simulink subsystem "electric_valva"  (R2022b)
settings: Solver=VariableStepAuto  StartTime=0.0  StopTime=10.0  RelTol=1e-3
values from neighbouring files (symbols this model uses):
  K = 6    [valva_run.m]
  L = 0.005    [valva_run.m]
  R = 3    [valva_run.m]
undefined symbols (not defined in the file or in its folder): magnitude
settings Model: Creator=rus_d  LastModifiedBy=rus_d

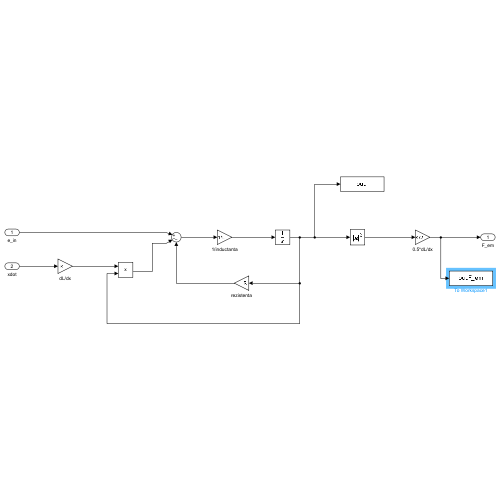
[thumbnail: Simulink's stored preview of the top-level diagram]
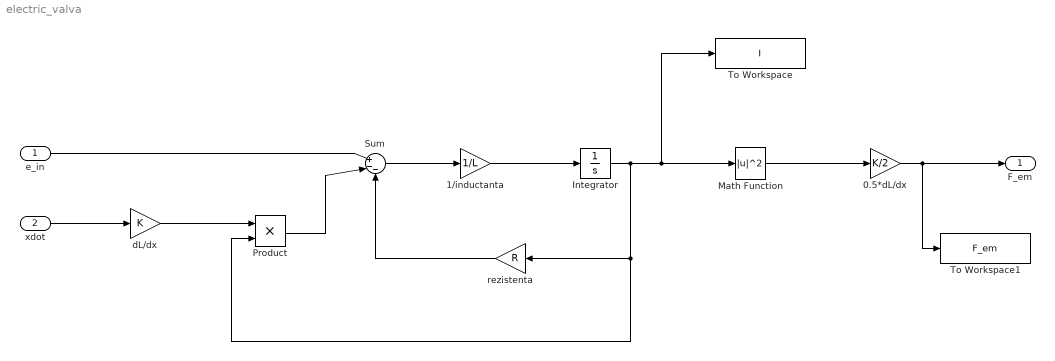
== system electric_valva ==
  e_in : Inport
  xdot : Inport  Port=2
  0.5*dL/dx : Gain  Gain=K/2
  1/inductanta : Gain  Gain=1/L
  Integrator : Integrator
  Math Function : Math  Operator=magnitude^2
  Product : Product
  Sum : Sum  Inputs=|+--
  To Workspace : ToWorkspace  VariableName=I  SampleTime=-1
  To Workspace1 : ToWorkspace  VariableName=F_em  SampleTime=-1
  dL/dx : Gain  Gain=K
  rezistenta : Gain  Gain=R
  F_em : Outport
  wires:
  xdot/1 -> dL/dx/1
  dL/dx/1 -> Product/1
  e_in/1 -> Sum/1
  Product/1 -> Sum/2
  Sum/1 -> 1/inductanta/1
  1/inductanta/1 -> Integrator/1
  Integrator/1 -> rezistenta/1, Product/2, To Workspace/1, Math Function/1
  Math Function/1 -> 0.5*dL/dx/1
  0.5*dL/dx/1 -> F_em/1, To Workspace1/1
  rezistenta/1 -> Sum/3
